simulink model "aie_testbench"  (R2021a)
settings: Solver=VariableStepAuto  StartTime=0.0  StopTime=384  RelTol=1e-3
PostLoadFcn:
  | data_in = xmcVitisRead('data/input.txt', 'cint16');
  | golden_out = xmcVitisRead('data/golden.txt', 'int32');
StopFcn:
  | % plot(data_out - double(golden_out));
  | % title('Error between Reference Output and Simulated Output');
undefined symbols (not defined in the file): None, S, vsva2197, xcvc1902
libraries: aieBasic x4, aieUtilities x2, dspsrcs4 x1, vmcUtilities x1, aieDSP x1
settings Model: Creator=robg  LastModifiedBy=robg
settings DataIOCC: SaveOutput=off  SignalLogging=off  DSMLogging=off  SaveTime=off  ReturnWorkspaceOutputs=off

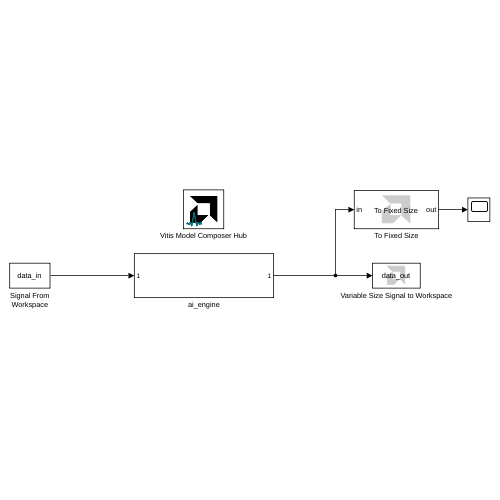
[thumbnail: Simulink's stored preview of the top-level diagram]
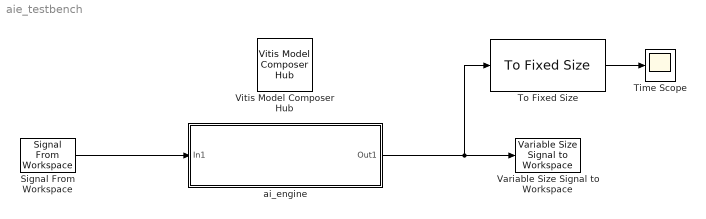
== system aie_testbench ==
  Signal From Workspace : dspsrcs4/Signal From Workspace  X=data_in  Ts=1  nsamps=128  OutputAfterFinalValue=Setting to zero  ignoreOrWarnInputAndFrameLengths=off  OutputFrames=off
  Time Scope : Scope
  To Fixed Size : aieUtilities/To Fixed Size  Mode=Stop simulation when input variable-size signal is not full  OutputSize=Inherit: Same as input  CopyMethod=Buffer samples to form output  HasStatusOutput=on
  Variable Size Signal to Workspace : aieUtilities/Variable Size Signal to Workspace  VariableNameMask=data_out
  Vitis Model Composer Hub : vmcUtilities/Vitis Model Composer Hub  Tag=genX  CodeGeneration=off  SubsystemName=ai_engine  TargetDirectory=./code_aie  ExportType=AI Engines  IpVendor=xilinx.com  IpLibrary=hls  IpVersion=1.0  IpHWLanguage=Verilog  AieCompilerOptions={}  AieSimulatorOptions={}  CreateTestbench=on  TestbenchStackSize=10  RunRtlSim=off  RunCSim=off  RunAieSim=on  AieSimTimeout=50000  RunAieSimProfiling=off  LaunchVitisAnalyzer=off  PlotOutput=off  RunX86Sim=off  X86SimTimeout=10  GenHwImage=off  GenLibadfXo=off  PlatformType=Specify Platform  Platform=/proj/xbuilds/SWIP/2023.2_1013_0023/installs/lin64/Vitis/2023.2/base_platforms/xilinx_vck190_base_202320_1/xilinx_vck190_base_202320_1.xpfm  HwSystemType=Baremetal  HwValidationTarget=hw  ProjDevice=Versal VCK190 Evaluation Platform (xcvc1902-vsva2197-2MP-e-S)  ProjDevicePart=xcvc1902-vsva2197-2MP-e-S  AIEType=AIE  SamplePeriod=-1  ClockFrequency=200  DataPathParallelism=1  xilinxfamily=versalaicore  part=xcvc1902  speed=-2MP-e-S  package=vsva2197  directory=./netlist  testbench=off  incr_netlist=off  synthesis_tool=Vivado  clock_wrapper=Clock Enables  dbl_ovrd=According to Block Masks  dcm_input_clock_period=10  sysclk_period=10  simulink_period=1  eval_field=0  IPInfoJsonString="{\"AIESubsystem\":{\"SubsystemName\":\"ai_engine\",\"TargetDirectory\":\"./code_aie\",\"SubsystemDir\":\"./code_aie/ip/ai_engine\"}}"  LogFileName=/proj/xcoswmktg/robg/git/vmc_examples/Vitis_Model_Composer/Examples/AIENGINE/Export_to_Vitis/code_aie/model_composer.log  NThreads=4
  ai_engine : Subsystem
  wires:
  To Fixed Size/1 -> Time Scope/1
  ai_engine/1(Out1) -> To Fixed Size/1, Variable Size Signal to Workspace/1
  Signal From Workspace/1 -> ai_engine/1(In1)

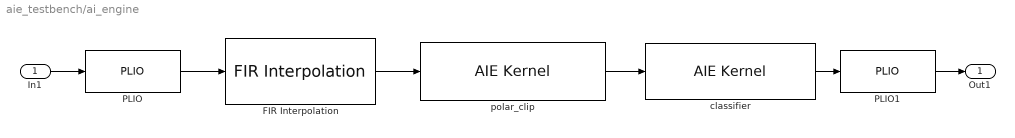
== system aie_testbench/ai_engine ==
  In1 : Inport
  FIR Interpolation : aieDSP/FIR Interpolation  data_type=cint16  coef_type=int16  use_coeff_reload=off  num_outputs=off  coeff=[33, -158, 0, 0, 491, -1214, 2674, 0, 0, -5942, 20503, 32767, 0, 0, 0, 0]  fir_length=32  interpolate_factor=2  input_window_size=128  shift_val=15  rnd_mode=Round to positive infinity  sat_mode=0-None  interp_poly=1  casc_length=1  blockJsonConstraints=[]  blockJsonConstraintsInternal=[]  spec=vmc_fir_interpolate_asym.json  SerializedMaskParamNames=[]  SerializedMaskParamValues=[]  SerializedMaskParamVisibilities=[]  block_type=FIR Interpolation  SerializedMaskParamDataypes=typename|typename|bool|bool|coef_type|uint|uint|uint|uint|uint|uint|uint|uint  SerializedMaskParamEnumStrArr=0|0|0|0|0|0|0|0|0|Floor,Ceiling,Round to positive infinity,Round to negative infinity,Round symmetrical to infinity,Round symmetrical to zero,Round convergent to even,Round convergent to odd|0-None,1-Asymmetric,3-Symmetric|0|0  SerializedMaskParamEnumValArr=0|0|0|0|0|0|0|0|0|0,1,2,3,4,5,6,7|0,1,3|0|0  SerializedMaskParamVectorArr=0|0|0|0|1|0|0|0|0|0|0|0|0
  PLIO : aieBasic/PLIO  PlioWidth=128  PlioFreqSpec=off  PlioFreq=250  ColLocation=0  channel=0  blockJsonConstraints=[]  deprecateConstraints=0
  PLIO1 : aieBasic/PLIO  PlioWidth=128  PlioFreqSpec=off  PlioFreq=250  ColLocation=0  channel=0  blockJsonConstraints=[]  deprecateConstraints=0
  classifier : aieBasic/AIE Kernel  KernelAllAttrs=s[12;12;9;9;19;14;21;23;21;23;24;21;15;17;12;24;26;26;26;27;28;9;21;23;23;23;24;25;14;19;19;29]@FunctionNameDeclFileNamePortNamesPortTypesPortSerializedTypesPortDirectionsPortWindowSizeEnablesPortWindowMarginEnablesPortBufferSizeEnablesPortBufferMarginEnablesPortSynchronicityEnablesPortSignalSizeEnablesPortBufferSizesPortBufferMarginsFunctionDeclFunctionTemplateSpecKindFunctionTemplateParamNamesFunctionTemplateParamKindsFunctionTemplateParamTypesFunctionTemplateParamValuesFunctionTemplateParamEnablesClassDeclClassTemplateSpecKindClassTemplateParamNamesClassTemplateParamKindsClassTemplateParamTypesClassTemplateParamValuesClassTemplateParamEnablesClassCtorDeclsClassCtorParamNamesClassCtorParamTypesClassCtorParamSerializedTypes[1 1]@C[32 1]@t10@classifiert19@../../aie/kernels.hC[2 1]@t5@inputt6@outputC[2 1]@t21@input_stream_cint16 *t38@adf::output_buffer< int32 > & restrictC[2 1]@t33@{P{Tinput_stream{1{t{Scint16}}}}}t40@{Q2{R{Tadf::output_buffer{1{t{Bi32}}}}}}C[2 1]@t5@inputt6@outputC[2 1]@l0@l1@C[2 1]@l0@l0@C[2 1]@l0@l1@C[2 1]@l0@l0@C[2 1]@l0@l1@C[2 1]@l0@l0@C[2 1]@nnC[2 1]@nnt91@void classifier(input_stream_cint16 * input, adf::output_buffer< int32 > & restrict output)t4@nonee[0 1]@e[0 1]@e[0 1]@e[0 1]@e[0 1]@nne[0 1]@e[0 1]@e[0 1]@e[0 1]@e[0 1]@e[0 1]@e[0 1]@e[0 1]@e[0 1]@  PortNames={'input'; 'output'}  PortSerializedTypes={'{P{Tinput_stream{1{t{Scint16}}}}}'; '{Q2{R{Tadf::output_buffer{1{t{Bi32}}}}}}'}  PortWindowSizes={0.000000000000000000e+00, 2.560000000000000000e+02}  PortWindowMargins={0.000000000000000000e+00, 0.000000000000000000e+00}  PortSynchronicities={'auto', 'sync'}  PortSignalSizes={0.000000000000000000e+00; 0.000000000000000000e+00}  FunctionTemplateSpecKind=none  FunctionTemplateParamNames={}  FunctionTemplateParamKinds={}  FunctionTemplateParamTypes={}  FunctionTemplateParamValues={}  FunctionIndex=1  FunctionTabVisible=on  FunctionTemplateParamsVisible=off  FunctionDeclTypeOptions=C[1 1]@t92@void classifier(input_stream_cint16 * input, adf::output_buffer< int32 > && restrict output)  FunctionDecl=void classifier(input_stream_cint16 * input, adf::output_buffer< int32 > && restrict output)  FunctionTemplateParams={}  FunctionTemplateParamsEnables={}  PortAttrs={ 'input', 'input', 'input_stream_cint16 *', '', '', '', ''; 'output', 'output', 'adf::output_buffer< int32 > & restrict', '256', '', 'sync', '' }  PortAttrsEnables={'off', 'off', 'off', 'off', 'off', 'off', 'off';'off', 'off', 'off', 'on', 'off', 'off', 'off'}  SampleTime=-1  KernelHeaderFile=aie/kernels.h  KernelFunction=classifier  KernelSourceFile=aie/kernels/classifiers/classify.cc  KernelSearchPaths={'./aie'}  PreProcOptions={}  blockJsonConstraints=[]
  polar_clip : aieBasic/AIE Kernel  KernelAllAttrs=s[12;12;9;9;19;14;21;23;21;23;24;21;15;17;12;24;26;26;26;27;28;9;21;23;23;23;24;25;14;19;19;29]@FunctionNameDeclFileNamePortNamesPortTypesPortSerializedTypesPortDirectionsPortWindowSizeEnablesPortWindowMarginEnablesPortBufferSizeEnablesPortBufferMarginEnablesPortSynchronicityEnablesPortSignalSizeEnablesPortBufferSizesPortBufferMarginsFunctionDeclFunctionTemplateSpecKindFunctionTemplateParamNamesFunctionTemplateParamKindsFunctionTemplateParamTypesFunctionTemplateParamValuesFunctionTemplateParamEnablesClassDeclClassTemplateSpecKindClassTemplateParamNamesClassTemplateParamKindsClassTemplateParamTypesClassTemplateParamValuesClassTemplateParamEnablesClassCtorDeclsClassCtorParamNamesClassCtorParamTypesClassCtorParamSerializedTypes[1 1]@C[32 1]@t10@polar_clipt19@../../aie/kernels.hC[2 1]@t2@int3@outC[2 1]@t21@input_stream_cint16 *t22@output_stream_cint16 *C[2 1]@t33@{P{Tinput_stream{1{t{Scint16}}}}}t34@{P{Toutput_stream{1{t{Scint16}}}}}C[2 1]@t5@inputt6@outputC[2 1]@l0@l0@C[2 1]@l0@l0@C[2 1]@l0@l0@C[2 1]@l0@l0@C[2 1]@l0@l0@C[2 1]@l0@l1@C[2 1]@nnC[2 1]@nnt69@void polar_clip(input_stream_cint16 * in, output_stream_cint16 * out)t4@nonee[0 1]@e[0 1]@e[0 1]@e[0 1]@e[0 1]@nne[0 1]@e[0 1]@e[0 1]@e[0 1]@e[0 1]@e[0 1]@e[0 1]@e[0 1]@e[0 1]@  PortNames={'in'; 'out'}  PortSerializedTypes={'{P{Tinput_stream{1{t{Scint16}}}}}'; '{P{Toutput_stream{1{t{Scint16}}}}}'}  PortWindowSizes={0.000000000000000000e+00, 0.000000000000000000e+00}  PortWindowMargins={0.000000000000000000e+00, 0.000000000000000000e+00}  PortSynchronicities={'auto', 'auto'}  PortSignalSizes={0.000000000000000000e+00; 2.560000000000000000e+02}  FunctionTemplateSpecKind=none  FunctionTemplateParamNames={}  FunctionTemplateParamKinds={}  FunctionTemplateParamTypes={}  FunctionTemplateParamValues={}  FunctionIndex=1  FunctionTabVisible=on  FunctionTemplateParamsVisible=off  FunctionDeclTypeOptions=C[1 1]@t69@void polar_clip(input_stream_cint16 * in, output_stream_cint16 * out)  FunctionDecl=void polar_clip(input_stream_cint16 * in, output_stream_cint16 * out)  FunctionTemplateParams={}  FunctionTemplateParamsEnables={}  PortAttrs={ 'input', 'in', 'input_stream_cint16 *', '', '', '', ''; 'output', 'out', 'output_stream_cint16 *', '', '', '', '256' }  PortAttrsEnables={'off', 'off', 'off', 'off', 'off', 'off', 'off';'off', 'off', 'off', 'off', 'off', 'off', 'on'}  SampleTime=-1  KernelHeaderFile=aie/kernels.h  KernelFunction=polar_clip  KernelSourceFile=aie/kernels/polar_clip.cpp  KernelSearchPaths={'./aie'}  PreProcOptions={}  blockJsonConstraints=[]
  Out1 : Outport
  wires:
  polar_clip/1 -> classifier/1
  FIR Interpolation/1 -> polar_clip/1
  classifier/1 -> PLIO1/1
  In1/1 -> PLIO/1
  PLIO/1 -> FIR Interpolation/1
  PLIO1/1 -> Out1/1
